simulink model "ExtendedKalmanFilter_model"  (R2015a)
settings: Solver=FixedStepDiscrete  StartTime=0.0  StopTime=10.0  FixedStep=parameters.dSamplingPeriod  RelTol=1e-3
InitFcn:
  | ExtendedKalmanFilter_config;
settings Model: Creator=hamada  LastModifiedBy=hamada

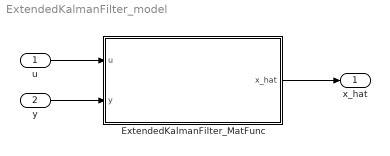
== system ExtendedKalmanFilter_model ==
  u : Inport  PortDimensions=3
  y : Inport  Port=2  PortDimensions=3
  ExtendedKalmanFilter_MatFunc : MATLAB Function  TreatAsAtomicUnit=on
  x_hat : Outport
  wires:
  u/1 -> ExtendedKalmanFilter_MatFunc/1(u)
  y/1 -> ExtendedKalmanFilter_MatFunc/2(y)
  ExtendedKalmanFilter_MatFunc/1(x_hat) -> x_hat/1

== matlab function ExtendedKalmanFilter_model/ExtendedKalmanFilter_MatFunc ==
  settings: sampleTime=parameters.dSamplingPeriod
  data: x_hat output double size=parameters.stateSize; u input double size=parameters.inputSize; y input double size=parameters.outputSize; parameters parameter
function x_hat = ExtendedKalmanFilter_MatFunc( u, y, parameters )
    %#codegen
    x_hat = ExtendedKalmanFilter( u, y, parameters );
end
